simulink model "codegen_drive"  (R2025b)
settings: Solver=FixedStepAuto  StartTime=0.0  StopTime=10  FixedStep=0.001  MaxStep=0.001  MinStep=0.001  RelTol=1e-3
model workspace (MAT data in the model file):
  L = 0.57
  La = 0.000279
  Ra = 0.288
  ahead = 0.75
  d = 0.74
  maxrpm = 6000
  pathx = Simulink.Parameter
  pathx.Complexity = 'real'
  pathx.Dimensions = [15 1]
  pathx.DataType = 'auto'
  pathy = Simulink.Parameter
  pathy.Complexity = 'real'
  pathy.Dimensions = [15 1]
  pathy.DataType = 'auto'
  rover_accel = 0.5
  roveracc = 0.5
  stepangle = 1.8
  w_r = 0.1
  wheelbase = 1
libraries: slpidlib x6
settings Model: Creator=egeda  LastModifiedBy=rowan
settings SolverCC: InitialStep=0.001
settings OptimizationCC: DefaultParameterBehavior=Inlined  UseDivisionForNetSlopeComputation=on  GainParamInheritBuiltInType=on  UseFloatMulNetSlope=on  InlineInvariantSignals=on  PassReuseOutputArgsAs=Individual arguments  ZeroExternalMemoryAtStartup=off  ZeroInternalMemoryAtStartup=off  NoFixptDivByZeroProtection=on  EfficientFloat2IntCast=on  LifeSpan=1  OptimizeBlockOrder=speed  DifferentSizesBufferReuse=on  EfficientTunableParamExpr=on
settings DebuggingCC: ParameterTunabilityLossMsg=error
settings HardwareCC: ProdBitPerInt=16.0  ProdBitPerPointer=16.0  ProdBitPerSizeT=16.0  ProdBitPerPtrDiffT=16.0  ProdLargestAtomicFloat=None  ProdWordSize=16.0  ProdLongLongMode=on  ProdHWDeviceType=STMicroelectronics->ST10/Super10
settings SFSimCC: MATLABDynamicMemAlloc=off
settings RTWCC: SystemTargetFile=ert.tlc  TemplateMakefile=ert_default_tmf  BuildConfiguration=Faster Runs  Description=Embedded Coder
settings CodeAppCC: ForceParamTrailComments=on  IgnoreCustomStorageClasses=off  OperatorAnnotations=on  SimulinkDataObjDesc=on  SFDataObjDesc=on  CustomSymbolStrGlobalVar=rt$N$M  CustomSymbolStrType=$N$M  CustomSymbolStrFcn=$N$M$F  CustomSymbolStrMacro=$N$M  InsertBlockDesc=on
settings ERTTargetCC: ERTCustomFileTemplate=example_file_process.tlc  ERTFilePackagingFormat=CompactWithDataFile  TargetLangStandard=C99 (ISO)  GenerateSampleERTMain=on  IncludeMdlTerminateFcn=off  CombineSignalStateStructs=on  SupportAbsoluteTime=off  SupportComplex=off  SupportNonInlinedSFcns=on

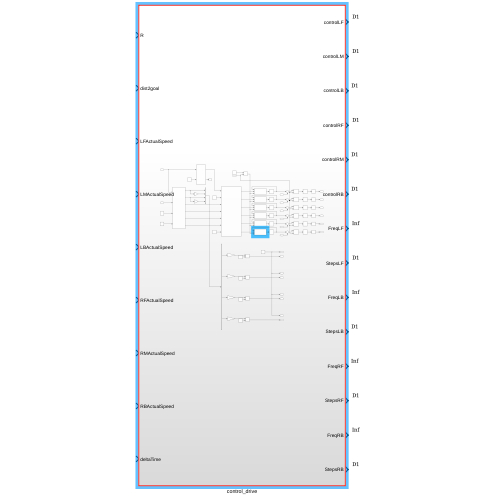
[thumbnail: Simulink's stored preview of the top-level diagram]
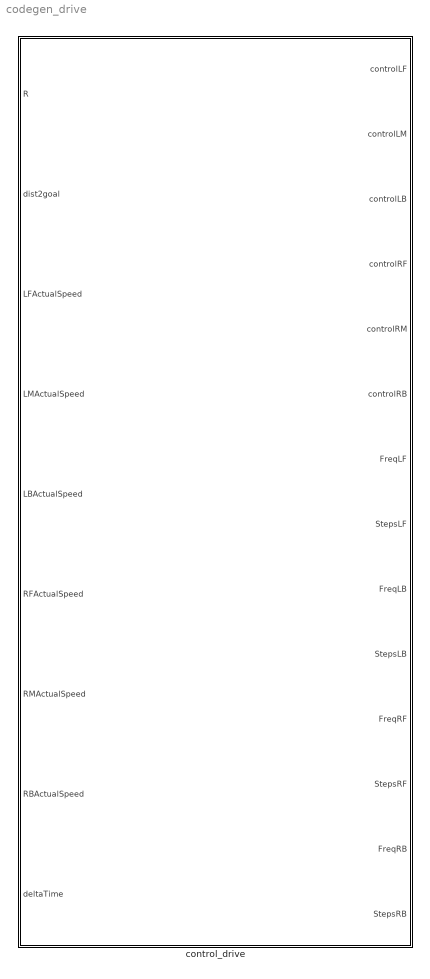
== system codegen_drive ==
  control_drive : Subsystem

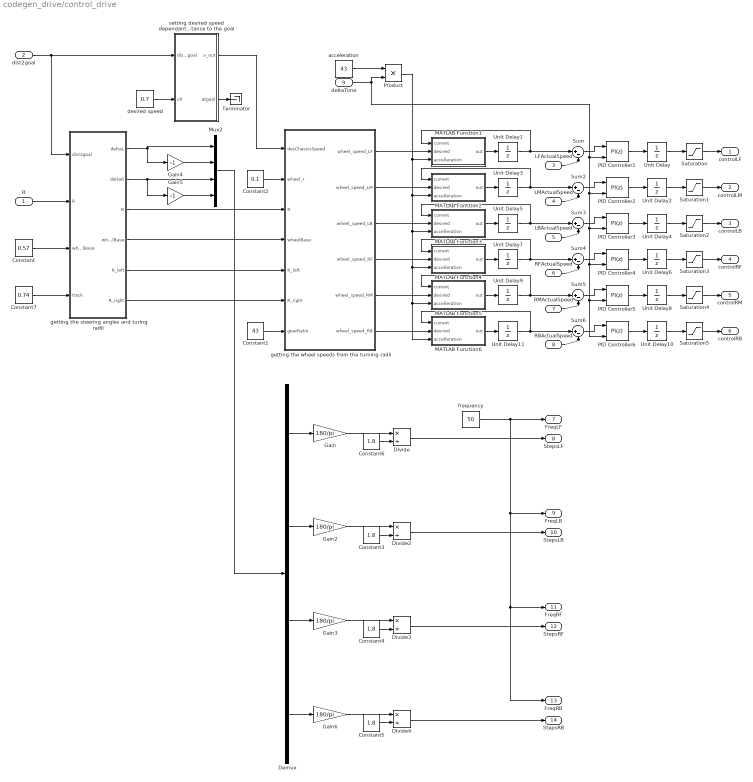
== system codegen_drive/control_drive ==
  R : Inport
  dist2goal : Inport  Port=2
  LFActualSpeed : Inport  Port=3
  LMActualSpeed : Inport  Port=4
  LBActualSpeed : Inport  Port=5
  RFActualSpeed : Inport  Port=6
  RMActualSpeed : Inport  Port=7
  RBActualSpeed : Inport  Port=8
  deltaTime : Inport  Port=9
  Constant : Constant  Value=0.57
  Constant1 : Constant  Value=43
  Constant2 : Constant  Value=0.1
  Constant{3..6} (4 alike) : Constant  Value=1.8
  Constant7 : Constant  Value=0.74
  Demux : Demux
  Divide{,2..4} (4 alike) : Product  Inputs=*/
  Gain{,2..3,6} (4 alike) : Gain  Gain=180/pi
  Gain4 : Gain  Gain=-1
  Gain5 : Gain  Gain=-1
  MATLAB Function1 : MATLAB Function  TreatAsAtomicUnit=on
  MATLAB Function2 : MATLAB Function  TreatAsAtomicUnit=on
  MATLAB Function3 : MATLAB Function  TreatAsAtomicUnit=on
  MATLAB Function4 : MATLAB Function  TreatAsAtomicUnit=on
  MATLAB Function5 : MATLAB Function  TreatAsAtomicUnit=on
  MATLAB Function6 : MATLAB Function  TreatAsAtomicUnit=on
  Mux2 : Mux
  PID Controller{1..6} (6 alike) : slpidlib/PID Controller  Controller=PI  Form=Parallel  TimeDomain=Discrete-time  UseExternalTs=on  SampleTime=-1  IntegratorMethod=Forward Euler  FilterMethod=Forward Euler  ControllerParametersSource=internal  P=0.2  I=0.2  UseKiTs=off  D=0  UseExternalDerivativeSource=off  N=100  UseFilter=on  TunerSelectOption=Transfer Function Based (PID Tuner App)  InitialConditionSource=internal  InitialConditionForIntegrator=0  InitialConditionForFilter=0  DifferentiatorICPrevScaledInput=0  ExternalReset=none  TrackingMode=off  Kt=1  LimitOutput=off  SatLimitsSource=internal  UpperSaturationLimit=inf  LowerSaturationLimit=-inf  LinearizeAsGain=on  AntiWindupMode=none  Kb=1  LimitIntegrator=off  UpperIntegratorSaturationLimit=inf  LowerIntegratorSaturationLimit=-inf  POutMin=[]  POutMax=[]  IOutMin=[]  IOutMax=[]  DOutMin=[]  DOutMax=[]  NOutMin=[]  NOutMax=[]  SumOutMin=[]  SumOutMax=[]  SaturationOutMin=[]  SaturationOutMax=[]  PParamMin=[]  PParamMax=[]  IParamMin=[]  IParamMax=[]  DParamMin=[]  DParamMax=[]  NParamMin=[]  NParamMax=[]  KbParamMin=[]  KbParamMax=[]  KtParamMin=[]  KtParamMax=[]  KbOutMin=[]  KbOutMax=[]  KtOutMin=[]  KtOutMax=[]  IntegratorOutMin=[]  IntegratorOutMax=[]  FilterOutMin=[]  FilterOutMax=[]  SumI1OutMin=[]  SumI1OutMax=[]  SumI2OutMin=[]  SumI2OutMax=[]  SumI3OutMin=[]  SumI3OutMax=[]  SumI4OutMin=[]  SumI4OutMax=[]  SumDOutMin=[]  SumDOutMax=[]  DifferentiatorOutMin=[]  DifferentiatorOutMax=[]  FilterDiffOutCoefMin=[]  FilterDiffOutCoefMax=[]  ReciprocalOutMin=[]  ReciprocalOutMax=[]  SumDenOutMin=[]  SumDenOutMax=[]  SumNumOutMin=[]  SumNumOutMax=[]  DivideOutMin=[]  DivideOutMax=[]  UdiffTsProdOutMin=[]  UdiffTsProdOutMax=[]  NTsProdOutMin=[]  NTsProdOutMax=[]  UintegralTsProdOutMin=[]  UintegralTsProdOutMax=[]  UngainTsProdOutMin=[]  UngainTsProdOutMax=[]  ClampingZeroOutDataTypeStr=Inherit: Inherit via back propagation  ClampingZeroOutMin=[]  ClampingZeroOutMax=[]  FilterDenConstantOutDataTypeStr=Inherit: Inherit via back propagation  FilterDenConstantOutMin=[]  FilterDenConstantOutMax=[]  PCopyOutDataTypeStr=Inherit: Inherit via back propagation  PCopyOutMin=[]  PCopyOutMax=[]  NCopyOutDataTypeStr=Inherit: Inherit via back propagation  NCopyOutMin=[]  NCopyOutMax=[]  IntegratorContinuousStateAttributes=''  IntegratorStateMustResolveToSignalObject=off  IntegratorRTWStateStorageClass=Auto  FilterContinuousStateAttributes=''  FilterStateMustResolveToSignalObject=off  FilterRTWStateStorageClass=Auto  ParallelPVariant=InternalParameters  IdealPVariant=Disabled  IVariant=InternalParameters  DVariant=Disabled  IntegratorVariant=Discrete  SatVariant=Disabled  AWVariant=Passthrough  PCopyVariant=Disabled  TRVariant=Disabled  FdbkBlocksVariant=Forward  IdealPFdbkVariant=Disabled  SatFdbkVariant=Disabled  DerivativeFilterVariant=Disabled  NVariant=Disabled  NCopyVariant=Disabled_SignalSpec  FilterICVariant=Disabled  IntegratorICVariant=InternalICs  ExternalResetVariant=Disabled  TRSumVariant=Passthrough  SumFdbkVariant=Disabled  SumVariant=Sum_PI  TsampFilterVariant=InternalTs  TsampNgainVariant=Passthrough  TsampIntegralVariant=ExternalTs  ExternalSaturationOutDataTypeStr=Inherit: Same as second input  DerivativeSourceVariant=Disabled  PreIntVariant=InternalPreInt
  Product : Product
  Saturation{,1..5} (6 alike) : Saturate  UpperLimit=5  LowerLimit=-5
  Sum{,2..6} (6 alike) : Sum  Inputs=|+-
  Terminator : Terminator
  Unit Delay{,1..11} (12 alike) : UnitDelay  SampleTime=-1  HasFrameUpgradeWarning=on
  acceleration : Constant  Value=43
  desired speed : Constant  Value=0.7
  frequency : Constant  Value=50
  getting the steering angles and turing radii : MATLAB Function  TreatAsAtomicUnit=on
  getting the wheel speeds from the turning radii : MATLAB Function  TreatAsAtomicUnit=on
  setting desired speed dependant on the distance to the goal : MATLAB Function  TreatAsAtomicUnit=on
  controlLF : Outport
  controlLM : Outport  Port=2
  controlLB : Outport  Port=3
  controlRF : Outport  Port=4
  controlRM : Outport  Port=5
  controlRB : Outport  Port=6
  FreqLF : Outport  Port=7
  StepsLF : Outport  Port=8
  FreqLB : Outport  Port=9
  StepsLB : Outport  Port=10
  FreqRF : Outport  Port=11
  StepsRF : Outport  Port=12
  FreqRB : Outport  Port=13
  StepsRB : Outport  Port=14
  wires:
  MATLAB Function1/1(out) -> Unit Delay1/1
  getting the wheel speeds from the turning radii/3(wheel_speed_LB) -> MATLAB Function3/2(desired)
  getting the wheel speeds from the turning radii/4(wheel_speed_RF) -> MATLAB Function4/2(desired)
  Sum/1 -> PID Controller1/1
  getting the wheel speeds from the turning radii/6(wheel_speed_RB) -> MATLAB Function6/2(desired)
  getting the wheel speeds from the turning radii/1(wheel_speed_LF) -> MATLAB Function1/2(desired)
  Unit Delay/1 -> Saturation/1
  getting the wheel speeds from the turning radii/5(wheel_speed_RM) -> MATLAB Function5/2(desired)
  Mux2/1 -> Demux/1
  desired speed/1 -> setting desired speed dependant on the distance to the goal/2(v0)
  dist2goal/1 -> setting desired speed dependant on the distance to the goal/1(dist2goal), getting the steering angles and turing radii/1(dist2goal)
  setting desired speed dependant on the distance to the goal/1(v_out) -> getting the wheel speeds from the turning radii/1(desChassisSpeed)
  getting the steering angles and turing radii/6(R_right) -> getting the wheel speeds from the turning radii/6(R_right)
  getting the steering angles and turing radii/1(deltaL) -> Mux2/1, Gain4/1
  getting the steering angles and turing radii/4(wheelBase) -> getting the wheel speeds from the turning radii/4(wheelBase)
  Gain4/1 -> Mux2/2
  getting the steering angles and turing radii/5(R_left) -> getting the wheel speeds from the turning radii/5(R_left)
  getting the steering angles and turing radii/2(deltaR) -> Gain5/1, Mux2/3
  Gain5/1 -> Mux2/4
  getting the steering angles and turing radii/3(R) -> getting the wheel speeds from the turning radii/3(R)
  Constant2/1 -> getting the wheel speeds from the turning radii/2(wheel_r)
  R/1 -> getting the steering angles and turing radii/2("R ")
  Saturation/1 -> controlLF/1
  PID Controller1/1 -> Unit Delay/1
  LFActualSpeed/1 -> Sum/2
  Unit Delay1/1 -> MATLAB Function1/1(current), Sum/1
  setting desired speed dependant on the distance to the goal/2(atgoal) -> Terminator/1
  getting the wheel speeds from the turning radii/2(wheel_speed_LM) -> MATLAB Function2/2(desired)
  LMActualSpeed/1 -> Sum2/2
  Unit Delay3/1 -> MATLAB Function2/1(current), Sum2/1
  MATLAB Function2/1(out) -> Unit Delay3/1
  Sum2/1 -> PID Controller2/1
  PID Controller2/1 -> Unit Delay2/1
  Unit Delay2/1 -> Saturation1/1
  Saturation1/1 -> controlLM/1
  LBActualSpeed/1 -> Sum3/2
  Unit Delay5/1 -> MATLAB Function3/1(current), Sum3/1
  Sum3/1 -> PID Controller3/1
  MATLAB Function3/1(out) -> Unit Delay5/1
  PID Controller3/1 -> Unit Delay4/1
  Unit Delay4/1 -> Saturation2/1
  Saturation2/1 -> controlLB/1
  RFActualSpeed/1 -> Sum4/2
  Unit Delay7/1 -> MATLAB Function4/1(current), Sum4/1
  Sum4/1 -> PID Controller4/1
  MATLAB Function4/1(out) -> Unit Delay7/1
  PID Controller4/1 -> Unit Delay6/1
  Unit Delay6/1 -> Saturation3/1
  Saturation3/1 -> controlRF/1
  RMActualSpeed/1 -> Sum5/2
  Unit Delay9/1 -> MATLAB Function5/1(current), Sum5/1
  Sum5/1 -> PID Controller5/1
  MATLAB Function5/1(out) -> Unit Delay9/1
  PID Controller5/1 -> Unit Delay8/1
  Unit Delay8/1 -> Saturation4/1
  Saturation4/1 -> controlRM/1
  RBActualSpeed/1 -> Sum6/2
  Unit Delay11/1 -> MATLAB Function6/1(current), Sum6/1
  Sum6/1 -> PID Controller6/1
  MATLAB Function6/1(out) -> Unit Delay11/1
  PID Controller6/1 -> Unit Delay10/1
  Unit Delay10/1 -> Saturation5/1
  Saturation5/1 -> controlRB/1
  Product/1 -> MATLAB Function4/3(accelleration), MATLAB Function5/3(accelleration), MATLAB Function6/3(accelleration), MATLAB Function3/3(accelleration), MATLAB Function2/3(accelleration), MATLAB Function1/3(accelleration)
  acceleration/1 -> Product/1
  deltaTime/1 -> Product/2, PID Controller4/2, PID Controller5/2, PID Controller6/2, PID Controller3/2, PID Controller2/2, PID Controller1/2
  Demux/1 -> Gain/1
  Gain/1 -> Divide/1
  Constant6/1 -> Divide/2
  Divide/1 -> StepsLF/1
  Divide2/1 -> StepsLB/1
  frequency/1 -> FreqRB/1, FreqRF/1, FreqLB/1, FreqLF/1
  Constant3/1 -> Divide2/2
  Gain2/1 -> Divide2/1
  Demux/2 -> Gain2/1
  Demux/3 -> Gain3/1
  Gain3/1 -> Divide3/1
  Constant4/1 -> Divide3/2
  Divide3/1 -> StepsRF/1
  Divide4/1 -> StepsRB/1
  Constant5/1 -> Divide4/2
  Gain6/1 -> Divide4/1
  Demux/4 -> Gain6/1
  Constant/1 -> getting the steering angles and turing radii/3("wheelBase ")
  Constant1/1 -> getting the wheel speeds from the turning radii/7(gearRatio)
  Constant7/1 -> getting the steering angles and turing radii/4(track)

== matlab function codegen_drive/control_drive/setting desired speed dependant on the distance to the goal ==
  data: dist2goal input; v0 input; v_out output; atgoal output
function [v_out, atgoal] = speed(dist2goal, v0)

%slow down if close to goal
if dist2goal <= 1
    v_out = 0;
    atgoal = 1;

%stopping if the rover is close to the target
elseif dist2goal <= 2
    v_out = v0 * 0.5;
    atgoal = 0;

%keeping cruising speed if not close to goal
else
    v_out = v0;
    atgoal = 0;
end

== matlab function codegen_drive/control_drive/MATLAB Function1 ==
  data: current input; out output; desired input; accelleration input
function out = linear_interpolation(current, desired, accelleration)
if current < desired
    current = current + accelleration;
end
if current > desired
    current = current - accelleration;
end

out = current;

== matlab function codegen_drive/control_drive/MATLAB Function2 ==
  data: current input; out output; desired input; accelleration input
function out = linear_interpolation(current, desired, accelleration)
if current < desired
    current = current + accelleration;
end
if current > desired
    current = current - accelleration;
end

out = current;

== matlab function codegen_drive/control_drive/MATLAB Function3 ==
  data: current input; out output; desired input; accelleration input
function out = linear_interpolation(current, desired, accelleration)
if current < desired
    current = current + accelleration;
end
if current > desired
    current = current - accelleration;
end

out = current;

== matlab function codegen_drive/control_drive/MATLAB Function4 ==
  data: current input; out output; desired input; accelleration input
function out = linear_interpolation(current, desired, accelleration)
if current < desired
    current = current + accelleration;
end
if current > desired
    current = current - accelleration;
end

out = current;

== matlab function codegen_drive/control_drive/MATLAB Function5 ==
  data: current input; out output; desired input; accelleration input
function out = linear_interpolation(current, desired, accelleration)
if current < desired
    current = current + accelleration;
end
if current > desired
    current = current - accelleration;
end

out = current;

== matlab function codegen_drive/control_drive/MATLAB Function6 ==
  data: current input; out output; desired input; accelleration input
function out = linear_interpolation(current, desired, accelleration)
if current < desired
    current = current + accelleration;
end
if current > desired
    current = current - accelleration;
end

out = current;

== matlab function codegen_drive/control_drive/getting the steering angles and turing radii ==
  data: dist2goal input; R input; deltaL output; deltaR output; R output; wheelBase output; R_left output; R_right output; wheelBase input; track input
function [deltaL,deltaR,R,wheelBase,R_left,R_right] = ackermann_angles(dist2goal,R,wheelBase,track)
    % Function to compute ackerman steering angles from a bicycle steer angle.
    if R == 0
        alpha = 0;
    else
        alpha = dist2goal/R;
    end
    
    R = abs(R);
    
    if alpha < 0
        R_left = (R+track/2);
        R_right = (R-track/2);
        deltaL = atan(wheelBase/(R_left));
        deltaR = atan(wheelBase/(R_right));
    elseif alpha > 0
        R_left = (R-track/2);
        R_right = (R+track/2);
        deltaL = -atan(wheelBase/(R_left));
        deltaR = -atan(wheelBase/(R_right));
    else
        deltaL = 0;
        deltaR = 0;
        R_left = R;
        R_right = R;
    end

end

== matlab function codegen_drive/control_drive/getting the wheel speeds from the turning radii ==
  data: desChassisSpeed input; wheel_speed_LF output; wheel_r input; R input; wheelBase input; R_left input; R_right input; wheel_speed_LM output; wheel_speed_LB output; wheel_speed_RF output; wheel_speed_RM output; wheel_speed_RB output; gearRatio input
function [wheel_speed_LF,wheel_speed_LM,wheel_speed_LB,wheel_speed_RF,wheel_speed_RM,wheel_speed_RB] = ...
          ackermann_speeds(desChassisSpeed,wheel_r,R,wheelBase,R_left,R_right,gearRatio)
if R > 0
    wheel_speed_LF = (desChassisSpeed/wheel_r)*sqrt(R_left^2 + (wheelBase/2)^2)/R;
    wheel_speed_LM = desChassisSpeed * R_left/(R*wheel_r);
    wheel_speed_LB = (desChassisSpeed/wheel_r)*sqrt(R_left^2 + (wheelBase/2)^2)/R;
    wheel_speed_RF = (desChassisSpeed/wheel_r)*sqrt(R_right^2 + (wheelBase/2)^2)/R;
    wheel_speed_RM = desChassisSpeed * R_right/(R*wheel_r);
    wheel_speed_RB = (desChassisSpeed/wheel_r)*sqrt(R_right^2 + (wheelBase/2)^2)/R;
else
    wheel_speed_LF = desChassisSpeed / wheel_r;
    wheel_speed_LM = desChassisSpeed / wheel_r;
    wheel_speed_LB = desChassisSpeed / wheel_r;
    wheel_speed_RF = desChassisSpeed / wheel_r;
    wheel_speed_RM = desChassisSpeed / wheel_r;
    wheel_speed_RB = desChassisSpeed / wheel_r;
end
    wheel_speed_LF = wheel_speed_LF * gearRatio;
    wheel_speed_LM = wheel_speed_LM * gearRatio;
    wheel_speed_LB = wheel_speed_LB * gearRatio;
    wheel_speed_RF = wheel_speed_RF * gearRatio;
    wheel_speed_RM = wheel_speed_RM * gearRatio;
    wheel_speed_RB = wheel_speed_RB * gearRatio;
end
